simulink model "aeropendulo_malha_aberta"  (R2024b)
settings: Solver=ode1  StartTime=0.0  StopTime=30  FixedStep=0.001  RelTol=1e-3  EnableMultiTasking=on
libraries: arduinolib x2, simulink x1
settings Model: ExtModeTrigDuration=2  Creator=João Victor  LastModifiedBy=João Victor
settings SolverCC: InitialStep=0.02  AutoInsertRateTranBlk=on
settings OptimizationCC: EnhancedBackFolding=on  PassReuseOutputArgsAs=Individual arguments  ZeroExternalMemoryAtStartup=off  ZeroInternalMemoryAtStartup=off  MaxStackSize=64  OptimizeBlockOrder=speed  DifferentSizesBufferReuse=on  OptimizationCustomize=off  EfficientTunableParamExpr=on
settings DebuggingCC: ParameterTunabilityLossMsg=error
settings HardwareCC: ProdBitPerInt=16  ProdBitPerPointer=16  ProdBitPerSizeT=16  ProdBitPerPtrDiffT=16  ProdLargestAtomicFloat=None  ProdWordSize=8  ProdHWDeviceType=Atmel->AVR  UseEmbeddedCoderFeatures=off
settings SFSimCC: MATLABDynamicMemAlloc=off
settings RTWCC: Description=Embedded Coder  SystemTargetFile=ert.tlc  HardwareBoard=Arduino Uno  TemplateMakefile=ert_default_tmf  Toolchain=Arduino AVR  BuildConfiguration=Faster Runs
settings CodeAppCC: ForceParamTrailComments=on  IgnoreCustomStorageClasses=off  OperatorAnnotations=on  SimulinkDataObjDesc=on  SFDataObjDesc=on  InsertBlockDesc=on
settings ERTTargetCC: SupportContinuousTime=on  SupportNonInlinedSFcns=on  SupportVariableSizeSignals=on  ExtModeTransport=3  ExtModeStaticAlloc=on  ExtModeAutomaticAllocSize=off  ExtModeStaticAllocSize=250  ExtModeMexFile=ext_xcp  ExtModeIntrfLevel=Level2 - Open  InlinedParameterPlacement=Hierarchical

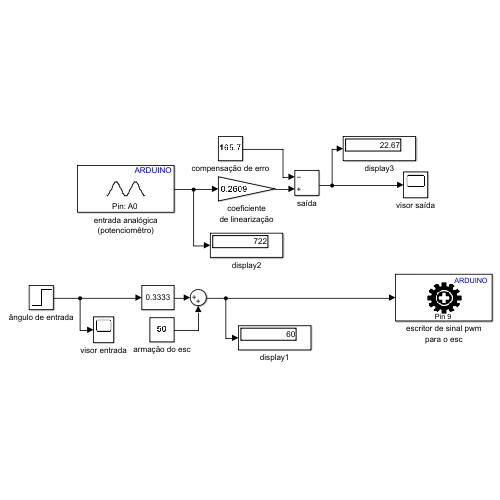
[thumbnail: Simulink's stored preview of the top-level diagram]
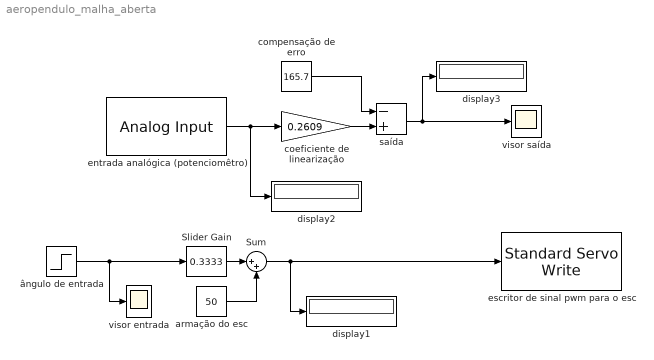
== system aeropendulo_malha_aberta ==
  Slider Gain : simulink/Math Operations/Slider Gain  gain=0.3333  low=0  high=255
  Sum : Sum  Inputs=|++
  armação do esc : Constant  Value=50
  coeficiente de linearização : Gain  Gain=0.2609
  compensação de erro : Constant  Value=165.7
  display1 : Display
  display2 : Display
  display3 : Display
  entrada analógica (potenciomêtro) : arduinolib/Analog Input  pinNumber=0  ReadResultsOnly=off  ConversionTriggerSource=Software  ExternalTriggerType=uint32( 0 )  OutputDataType=uint16  EnableConversionCompleteNotify=off  EnableOuputStatus=off  SampleTime=-1  blockPlatform=arduino
      settings: SourceProductName=Common
  escritor de sinal pwm para o esc : arduinolib/Standard Servo Write  pinNumber=9  ServoIndex=0  blockPlatform=ARDUINO
      settings: SourceProductName=Common
  saída : Sum  Inputs=-+
  visor entrada : Scope
  visor saída : Scope
  ângulo de entrada : Step  Time=5  After=30  SampleTime=0
  wires:
  compensação de erro/1 -> saída/1
  saída/1 -> display3/1, visor saída/1
  entrada analógica (potenciomêtro)/1 -> display2/1, coeficiente de linearização/1
  coeficiente de linearização/1 -> saída/2
  Sum/1 -> escritor de sinal pwm para o esc/1, display1/1
  Slider Gain/1 -> Sum/1
  armação do esc/1 -> Sum/2
  ângulo de entrada/1 -> Slider Gain/1, visor entrada/1
